simulink model "Model_2"  (R2018a)
settings: Solver=ode3  StartTime=0.0  StopTime=20  FixedStep=0.00001  RelTol=1e-3  EnableMultiTasking=on
values from neighbouring files (symbols this model uses):
  K = K(3:end,3:end)    [Etude_convergence_EF.m]
  M = M(3:end,3:end)    [Etude_convergence_EF.m]
undefined symbols (not defined in the file or in its folder): C, V0
settings Model: Creator=p202400  LastModifiedBy=sitanb
settings DataIOCC: LimitDataPoints=on  SaveFormat=Array  SignalLoggingSaveFormat=ModelDataLogs
settings OptimizationCC: ExpressionDepthLimit=2147483647  LifeSpan=inf
settings DebuggingCC: UnderspecifiedInitializationDetection=Classic  MergeDetectMultiDrivingBlocksExec=none  SolverPrmCheckMsg=warning  FcnCallInpInsideContextMsg=warning  StateNameClashWarn=warning  SFUnexpectedBacktrackingDiag=warning  SFNoUnconditionalDefaultTransitionDiag=warning  SFExecutionAtInitializationDiag=none
settings HardwareCC: ProdBitPerPointer=32  ProdBitPerSizeT=32  ProdBitPerPtrDiffT=32  ProdLargestAtomicFloat=None  ProdIntDivRoundTo=Undefined  ProdEndianess=Unspecified  ProdWordSize=32  ProdHWDeviceType=32-bit Generic
settings ModelReferenceCC: PropagateSignalLabelsOutOfModel=off
settings CodeAppCC: StateflowObjectComments=on
settings GRTTargetCC: TargetLangStandard=C89/C90 (ANSI)  GeneratePreprocessorConditionals=Disable all  CombineOutputUpdateFcns=off  GRTInterface=on
settings ConfigComp: CovMetricSettings=dw  CovHtmlReporting=on  CovSaveCumulativeToWorkspaceVar=on  CovSaveSingleToWorkspaceVar=on  CovExternalEMLEnable=off

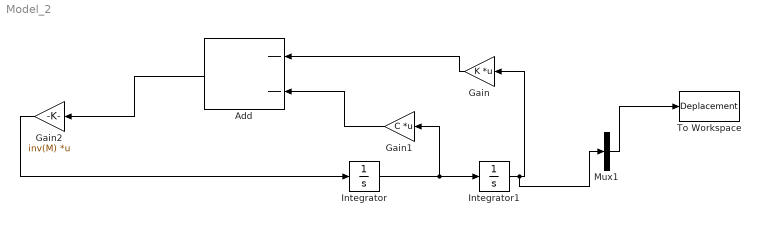
== system Model_2 ==
  Add : Sum  Inputs=--
  Gain : Gain  Gain=K  Multiplication=Matrix(K*u) (u vector)
  Gain1 : Gain  Gain=C  Multiplication=Matrix(K*u) (u vector)
  Gain2 : Gain  Gain=inv(M)  Multiplication=Matrix(K*u) (u vector)
  Integrator : Integrator  InitialCondition=V0
  Integrator1 : Integrator
  Mux1 : Mux  Inputs=1
  To Workspace : ToWorkspace  VariableName=Deplacement  SampleTime=-1
  wires:
  Integrator/1 -> Integrator1/1, Gain1/1
  Integrator1/1 -> Mux1/1, Gain/1
  Gain1/1 -> Add/2
  Gain/1 -> Add/1
  Mux1/1 -> To Workspace/1
  Gain2/1 -> Integrator/1
  Add/1 -> Gain2/1
